simulink model "stateSpaceSim"  (R2020b)
settings: Solver=FixedStepAuto  StartTime=0.0  StopTime=10  FixedStep=Ts  RelTol=1e-3
values from neighbouring files (symbols this model uses):
  Ao = Az    [CONTROLLO_STATE_SPACE.m]    (also in C_CONTROLLO_STATESPACE_AUG.m = [Az Bz; zeros(1,4) 1]; ControlloLQRStateSpace.m = [Az Bz; zeros(1,4) 1]; f_Obj_LQR.m = [Az Bz; zeros(1,4) 1])
  As = Ps.A    [C1_CONTROLLO_STATESPACE.m]    (also in CONTROLLO_STATE_SPACE.m; C_CONTROLLO_STATESPACE_AUG.m; ControlloLQRStateSpace.m; FminconOptim.m)
  Az = Pz.A    [C1_CONTROLLO_STATESPACE.m]    (also in CONTROLLO_STATE_SPACE.m; C_CONTROLLO_STATESPACE_AUG.m; ControlloLQRStateSpace.m; FminconOptim.m)
  Bo = Bz    [CONTROLLO_STATE_SPACE.m]    (also in C_CONTROLLO_STATESPACE_AUG.m = [Bz; 0]; ControlloLQRStateSpace.m = [Bz; 0]; f_Obj_LQR.m = [Bz; 0])
  Bs = Ps.B    [C1_CONTROLLO_STATESPACE.m]    (also in CONTROLLO_STATE_SPACE.m; C_CONTROLLO_STATESPACE_AUG.m; ControlloLQRStateSpace.m; FminconOptim.m)
  Bz = Pz.B    [C1_CONTROLLO_STATESPACE.m]    (also in CONTROLLO_STATE_SPACE.m; C_CONTROLLO_STATESPACE_AUG.m; ControlloLQRStateSpace.m; FminconOptim.m)
  Co = Cz    [CONTROLLO_STATE_SPACE.m]    (also in C_CONTROLLO_STATESPACE_AUG.m = [Cz 0]; ControlloLQRStateSpace.m = [Cz 0]; f_Obj_LQR.m = [Cz 0])
  Cs = Ps.C    [C1_CONTROLLO_STATESPACE.m]    (also in CONTROLLO_STATE_SPACE.m; C_CONTROLLO_STATESPACE_AUG.m; ControlloLQRStateSpace.m; FminconOptim.m)
  Cz = Pz.C    [C1_CONTROLLO_STATESPACE.m]    (also in CONTROLLO_STATE_SPACE.m; C_CONTROLLO_STATESPACE_AUG.m; ControlloLQRStateSpace.m; FminconOptim.m)
  H = -Khat(:,n+1:end)    [C1_CONTROLLO_STATESPACE.m]    (also in CONTROLLO_STATE_SPACE.m = - Khat(:, n+1:end); C_CONTROLLO_STATESPACE_AUG.m; ControlloLQRStateSpace.m; controllo_retroazione.m = 1)
  K = Khat(:,1:n)    [C1_CONTROLLO_STATESPACE.m]    (also in CONTROLLO_STATE_SPACE.m = Khat(:, 1:n); C_CONTROLLO_STATESPACE_AUG.m; ControlloLQRStateSpace.m; f_Obj_LQR.m)
  L = place(Az', Cz', Po_d(1:end-1))'    [C1_CONTROLLO_STATESPACE.m]    (also in CONTROLLO_CONTINUO.m = C*P; CONTROLLO_STATE_SPACE.m = place(Ao', Co', o(1:end-1))'; C_CONTROLLO_STATESPACE_AUG.m = place(Ao', Co', Po_d(1:end))'; ControlloLQRStateSpace.m = place(Ao', Co', Po_d(1:end))')
  Ts = system.getSamplingPeriod    [CONTROLLO_CONTINUO.m]    (also in IDENTIFICAZIONE.m; ID_multisine.m; ID_sinestream.m; controllo_ottimo.m)
  u_max = system.getUMax    [CONTROLLO_CONTINUO.m]    (also in IDENTIFICAZIONE.m; controllo_ottimo.m; controllo_retroazione.m; matlab.mat = 50)
undefined symbols (not defined in the file or in its folder): DiscIntNeverNeededParam
libraries: cstblocks x1
settings Model: Creator=miche  LastModifiedBy=miche

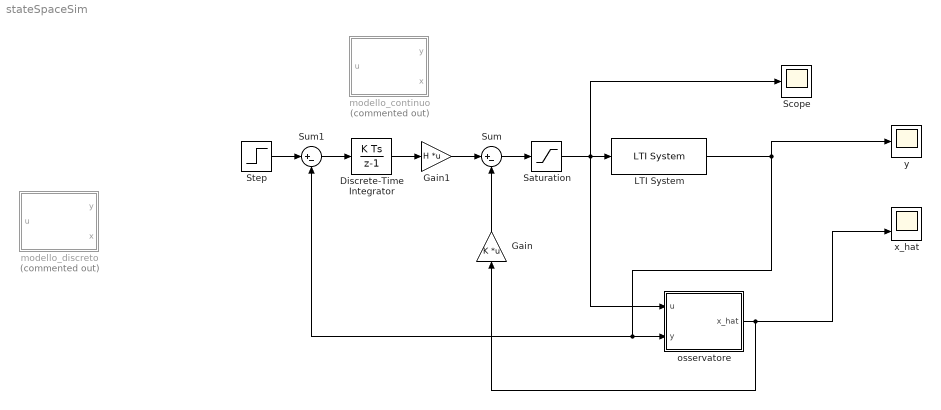
== system stateSpaceSim ==
  Discrete-Time Integrator : DiscreteIntegrator  gainval=1  SampleTime=Ts  ICPrevOutput=DiscIntNeverNeededParam  ICPrevScaledInput=DiscIntNeverNeededParam
  Gain : Gain  Gain=K  Multiplication=Matrix(K*u)
  Gain1 : Gain  Gain=H  Multiplication=Matrix(K*u)
  LTI System : cstblocks/LTI System  sys=Ps  IC=[]
  Saturation : Saturate  UpperLimit=u_max  LowerLimit=-u_max
  Scope : Scope
  Step : Step  Time=0  SampleTime=0
  Sum : Sum  Inputs=|+-
  Sum1 : Sum  Inputs=|+-
  modello_continuo : Subsystem  Commented=on
  modello_discreto : Subsystem  Commented=on
  osservatore : Subsystem
  x_hat : Scope  NumInputPorts=2
  y : Scope
  wires:
  osservatore/1(x_hat) -> x_hat/2, Gain/1
  Gain/1 -> Sum/2
  LTI System/1 -> y/1, Sum1/2, osservatore/2(y)
  Gain1/1 -> Sum/1
  Discrete-Time Integrator/1 -> Gain1/1
  Sum1/1 -> Discrete-Time Integrator/1
  Step/1 -> Sum1/1
  Sum/1 -> Saturation/1
  Saturation/1 -> osservatore/1(u), LTI System/1, Scope/1
  ? -> x_hat/1

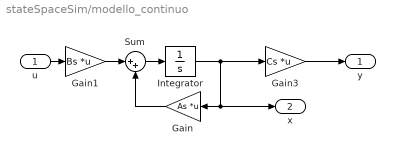
== system stateSpaceSim/modello_continuo ==
  u : Inport
  Gain : Gain  Gain=As  Multiplication=Matrix(K*u)
  Gain1 : Gain  Gain=Bs  Multiplication=Matrix(K*u)
  Gain3 : Gain  Gain=Cs  Multiplication=Matrix(K*u)
  Integrator : Integrator
  Sum : Sum  Inputs=|++
  y : Outport
  x : Outport  Port=2
  wires:
  Integrator/1 -> Gain/1, x/1, Gain3/1
  u/1 -> Gain1/1
  Gain3/1 -> y/1
  Gain/1 -> Sum/2
  Sum/1 -> Integrator/1
  Gain1/1 -> Sum/1

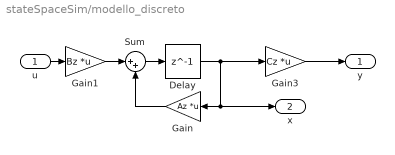
== system stateSpaceSim/modello_discreto ==
  u : Inport
  Delay : Delay  DelayLength=1
  Gain : Gain  Gain=Az  Multiplication=Matrix(K*u)
  Gain1 : Gain  Gain=Bz  Multiplication=Matrix(K*u)
  Gain3 : Gain  Gain=Cz  Multiplication=Matrix(K*u)
  Sum : Sum  Inputs=|++
  y : Outport
  x : Outport  Port=2
  wires:
  Delay/1 -> Gain/1, x/1, Gain3/1
  u/1 -> Gain1/1
  Gain3/1 -> y/1
  Gain/1 -> Sum/2
  Sum/1 -> Delay/1
  Gain1/1 -> Sum/1

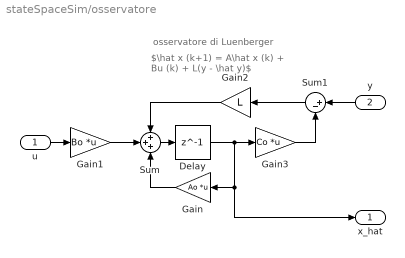
== system stateSpaceSim/osservatore ==
  note: osservatore di Luenberger
  note: $\hat x (k+1) = A\hat x (k) + Bu (k) + L(y - \hat y)$
  u : Inport
  y : Inport  Port=2
  Delay : Delay  DelayLength=1
  Gain : Gain  Gain=Ao  Multiplication=Matrix(K*u)
  Gain1 : Gain  Gain=Bo  Multiplication=Matrix(K*u)
  Gain2 : Gain  Gain=L
  Gain3 : Gain  Gain=Co  Multiplication=Matrix(K*u)
  Sum : Sum  Inputs=+++
  Sum1 : Sum  Inputs=|+-
  x_hat : Outport
  wires:
  Delay/1 -> x_hat/1, Gain/1, Gain3/1
  u/1 -> Gain1/1
  Gain3/1 -> Sum1/2
  Sum/1 -> Delay/1
  Gain1/1 -> Sum/2
  Gain/1 -> Sum/3
  y/1 -> Sum1/1
  Sum1/1 -> Gain2/1
  Gain2/1 -> Sum/1
